simulink model "zbiorniki_model"  (R2015a)
settings: Solver=ode45  StartTime=0.0  StopTime=2000  MaxStep=1  RelTol=1e-3
values from neighbouring files (symbols this model uses):
  sol1 = [39.7748134318 0.299881384341 23.9796211007]    [Parameters.mat]
  sol2 = [36.7179430006 0.289884578256 23.9243003658]    [Parameters.mat]
  sol3 = [25.2230732075 0.430131715234 24.0382421423]    [Parameters.mat]
settings Model: Creator=Student  LastModifiedBy=Student

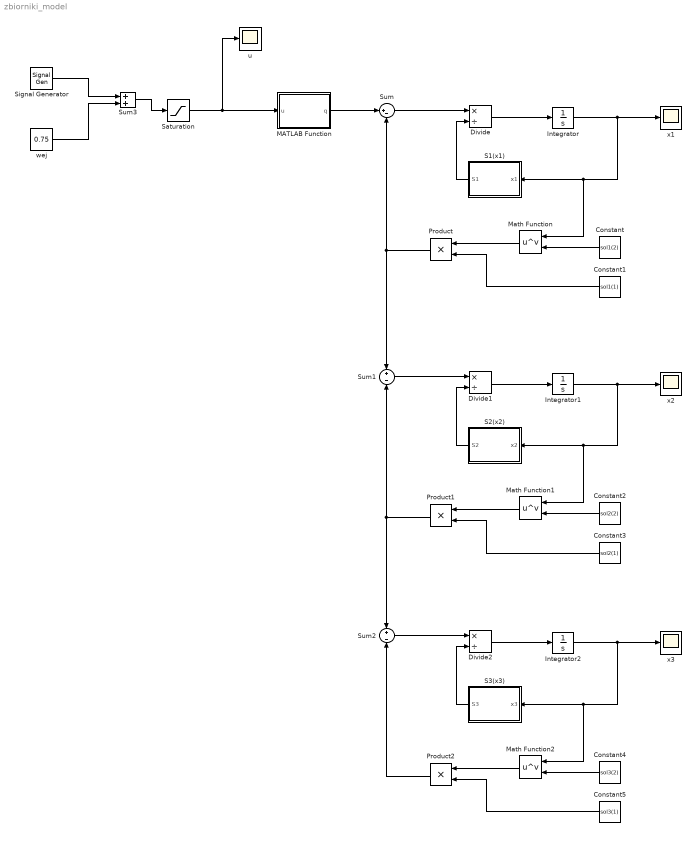
== system zbiorniki_model ==
  Constant : Constant  Value=sol1(2)
  Constant1 : Constant  Value=sol1(1)
  Constant2 : Constant  Value=sol2(2)
  Constant3 : Constant  Value=sol2(1)
  Constant4 : Constant  Value=sol3(2)
  Constant5 : Constant  Value=sol3(1)
  Divide : Product  Inputs=*/
  Divide1 : Product  Inputs=*/
  Divide2 : Product  Inputs=*/
  Integrator : Integrator  InitialCondition=10  LimitOutput=on  LowerSaturationLimit=0.1
  Integrator1 : Integrator  InitialCondition=10  LimitOutput=on  LowerSaturationLimit=0.1
  Integrator2 : Integrator  InitialCondition=10  LimitOutput=on  LowerSaturationLimit=0.1
  MATLAB Function : MATLAB Function  TreatAsAtomicUnit=on
  Math Function : Math  Operator=pow  SaturateOnIntegerOverflow=on
  Math Function1 : Math  Operator=pow  SaturateOnIntegerOverflow=on
  Math Function2 : Math  Operator=pow  SaturateOnIntegerOverflow=on
  Product : Product
  Product1 : Product
  Product2 : Product
  S1(x1) : MATLAB Function  TreatAsAtomicUnit=on
  S2(x2) : MATLAB Function  TreatAsAtomicUnit=on
  S3(x3) : MATLAB Function  TreatAsAtomicUnit=on
  Saturation : Saturate  UpperLimit=1  LowerLimit=0.5
  Signal Generator : SignalGenerator  WaveForm=square  Amplitude=0.2  Frequency=1/50
  Sum : Sum  Inputs=|+-
  Sum1 : Sum  Inputs=+-
  Sum2 : Sum  Inputs=+-
  Sum3 : Sum
  u : Scope
  wej : Constant  Value=0.75
  x1 : Scope
  x2 : Scope
      settings: SaveName=ScopeData2
  x3 : Scope
      settings: SaveName=ScopeData3
  wires:
  Saturation/1 -> MATLAB Function/1(u), u/1
  MATLAB Function/1(q) -> Sum/1
  Sum/1 -> Divide/1
  S1(x1)/1(S1) -> Divide/2
  Divide/1 -> Integrator/1
  Integrator/1 -> Math Function/1, S1(x1)/1(x1), x1/1
  Constant/1 -> Math Function/2
  Math Function/1 -> Product/1
  Constant1/1 -> Product/2
  Product/1 -> Sum/2, Sum1/1
  Sum1/1 -> Divide1/1
  S2(x2)/1(S2) -> Divide1/2
  Divide1/1 -> Integrator1/1
  Integrator1/1 -> Math Function1/1, S2(x2)/1(x2), x2/1
  Constant2/1 -> Math Function1/2
  Math Function1/1 -> Product1/1
  Constant3/1 -> Product1/2
  Product1/1 -> Sum2/1, Sum1/2
  Sum2/1 -> Divide2/1
  S3(x3)/1(S3) -> Divide2/2
  Divide2/1 -> Integrator2/1
  Integrator2/1 -> Math Function2/1, S3(x3)/1(x3), x3/1
  Constant4/1 -> Math Function2/2
  Math Function2/1 -> Product2/1
  Constant5/1 -> Product2/2
  Product2/1 -> Sum2/2
  Signal Generator/1 -> Sum3/1
  wej/1 -> Sum3/2
  Sum3/1 -> Saturation/1

== matlab function zbiorniki_model/S1(x1) ==
  data: x1 input; S1 output
function S1 = fcn(x1)
a = 10;
b = 44.5;
c = 25;
w = 3.5;
H = 35;
R = 36.4;
S1 = c*w;

== matlab function zbiorniki_model/MATLAB Function ==
  data: u input; q output
function q = fcn(u)
a = -231.6274;
b = 625.0864;
c = -254.4828;
q = a*(u^2) + b*u + c;

== matlab function zbiorniki_model/S2(x2) ==
  data: x2 input; S2 output
function S2 = fcn(x2)
a = 10;
b = 44.5;
c = 25;
w = 3.5;
H = 35;
R = 36.4;
S2 = w*(((b-a)/H)*x2 + a);

== matlab function zbiorniki_model/S3(x3) ==
  data: x3 input; S3 output
function S3 = fcn(x3)
a = 10;
b = 44.5;
c = 25;
w = 3.5;
H = 35;
R = 36.4;
S3 = w*sqrt(2*R*x3 - x3^2);
